simulink model "HillHold"  (R2022b)
settings: Solver=FixedStepDiscrete  StartTime=0.0  StopTime=10.0  FixedStep=0.0001  RelTol=1e-3
undefined symbols (not defined in the file or in its folder): GEAR, MOTORDIR, ParamCfg_HillholdEnable_u16, ParamCfg_HillHoldTime_u16
libraries: simulink x29
settings Model: DataDictionary=MCU_HillHold.sldd  Creator=ZYH  LastModifiedBy=ZYH
settings OptimizationCC: DefaultParameterBehavior=Inlined  EnhancedBackFolding=on  PassReuseOutputArgsAs=Individual arguments  ZeroExternalMemoryAtStartup=off  ZeroInternalMemoryAtStartup=off  OptimizeBlockOrder=speed  DifferentSizesBufferReuse=on  OptimizationCustomize=off  EfficientTunableParamExpr=on
settings DebuggingCC: ParameterTunabilityLossMsg=error
settings SFSimCC: MATLABDynamicMemAlloc=off
settings RTWCC: Description=Embedded Coder  SystemTargetFile=ert.tlc  GenCodeOnly=on  TemplateMakefile=ert_default_tmf
settings CodeAppCC: ForceParamTrailComments=on  IgnoreCustomStorageClasses=off  OperatorAnnotations=on  SimulinkDataObjDesc=on  SFDataObjDesc=on  InsertBlockDesc=on
settings ERTTargetCC: TargetLangStandard=C99 (ISO)  GenerateSampleERTMain=on  InlinedParameterPlacement=NonHierarchical  ERTCustomFileTemplate=example_file_process.tlc

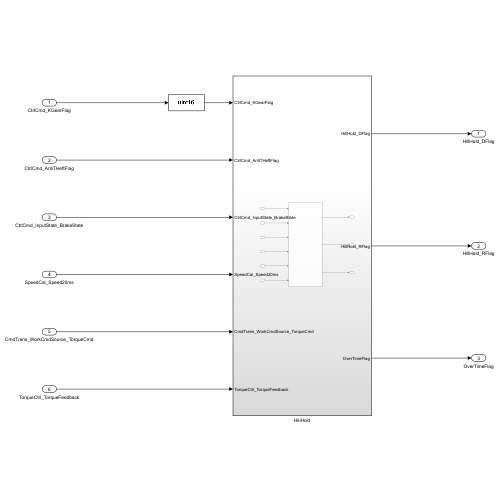
[thumbnail: Simulink's stored preview of the top-level diagram]
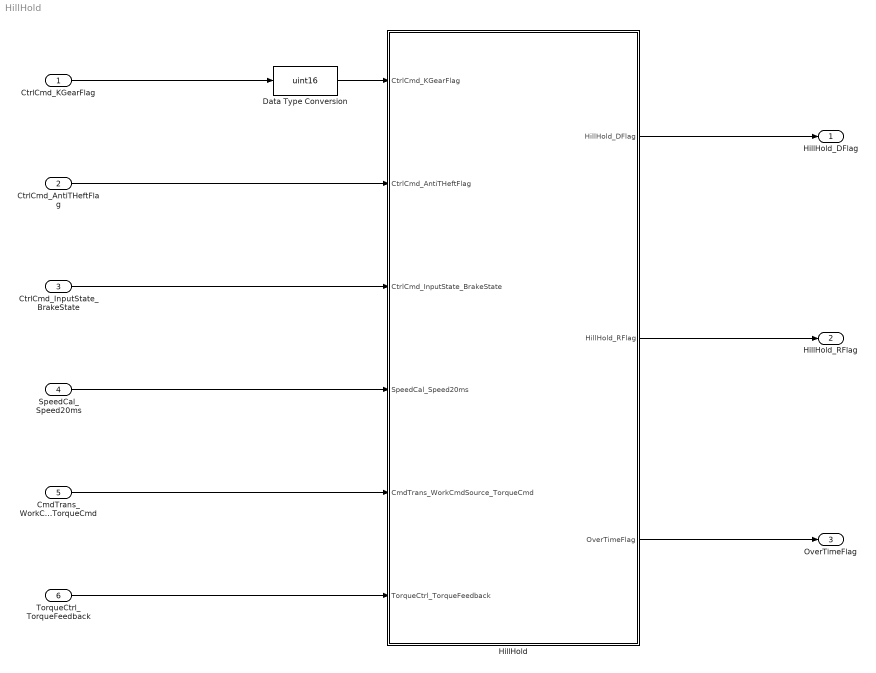
== system HillHold ==
  CtrlCmd_KGearFlag : Inport
  CtrlCmd_AntiTHeftFlag : Inport  Port=2
  CtrlCmd_InputState_BrakeState : Inport  Port=3
  SpeedCal_Speed20ms : Inport  Port=4
  CmdTrans_WorkCmdSource_TorqueCmd : Inport  Port=5
  TorqueCtrl_TorqueFeedback : Inport  Port=6
  Data Type Conversion : DataTypeConversion  OutDataTypeStr=uint16  SaturateOnIntegerOverflow=off  RndMeth=Floor
  HillHold : Subsystem
  HillHold_DFlag : Outport
  HillHold_RFlag : Outport  Port=2
  OverTimeFlag : Outport  Port=3
  wires:
  CtrlCmd_KGearFlag/1 -> Data Type Conversion/1
  CtrlCmd_AntiTHeftFlag/1 -> HillHold/2(CtrlCmd_AntiTHeftFlag)
  Data Type Conversion/1 -> HillHold/1(CtrlCmd_KGearFlag)
  CtrlCmd_InputState_BrakeState/1 -> HillHold/3(CtrlCmd_InputState_BrakeState)
  SpeedCal_Speed20ms/1 -> HillHold/4(SpeedCal_Speed20ms)
  CmdTrans_WorkCmdSource_TorqueCmd/1 -> HillHold/5(CmdTrans_WorkCmdSource_TorqueCmd)
  TorqueCtrl_TorqueFeedback/1 -> HillHold/6(TorqueCtrl_TorqueFeedback)
  HillHold/1(HillHold_DFlag) -> HillHold_DFlag/1
  HillHold/2(HillHold_RFlag) -> HillHold_RFlag/1
  HillHold/3(OverTimeFlag) -> OverTimeFlag/1

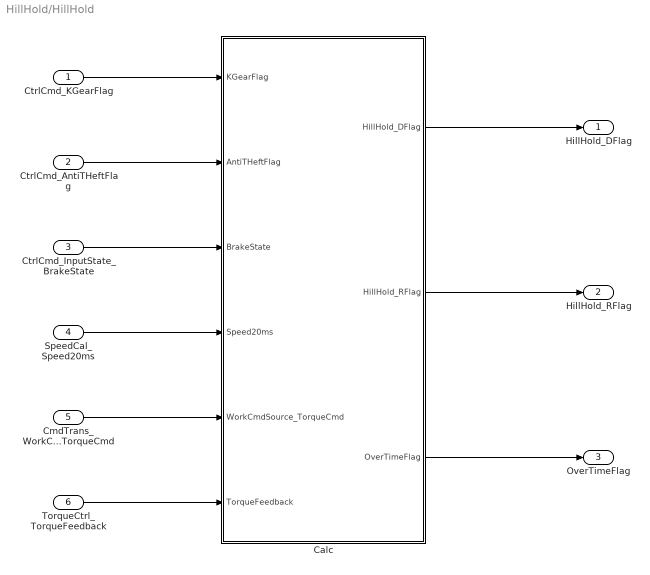
== system HillHold/HillHold ==
  CtrlCmd_KGearFlag : Inport
  CtrlCmd_AntiTHeftFlag : Inport  Port=2
  CtrlCmd_InputState_BrakeState : Inport  Port=3
  SpeedCal_Speed20ms : Inport  Port=4
  CmdTrans_WorkCmdSource_TorqueCmd : Inport  Port=5
  TorqueCtrl_TorqueFeedback : Inport  Port=6
  Calc : Subsystem
  HillHold_DFlag : Outport
  HillHold_RFlag : Outport  Port=2
  OverTimeFlag : Outport  Port=3
  wires:
  CtrlCmd_KGearFlag/1 -> Calc/1(KGearFlag)
  CtrlCmd_AntiTHeftFlag/1 -> Calc/2(AntiTHeftFlag)
  CtrlCmd_InputState_BrakeState/1 -> Calc/3(BrakeState)
  SpeedCal_Speed20ms/1 -> Calc/4(Speed20ms)
  CmdTrans_WorkCmdSource_TorqueCmd/1 -> Calc/5(WorkCmdSource_TorqueCmd)
  TorqueCtrl_TorqueFeedback/1 -> Calc/6(TorqueFeedback)
  Calc/1(HillHold_DFlag) -> HillHold_DFlag/1
  Calc/2(HillHold_RFlag) -> HillHold_RFlag/1
  Calc/3(OverTimeFlag) -> OverTimeFlag/1

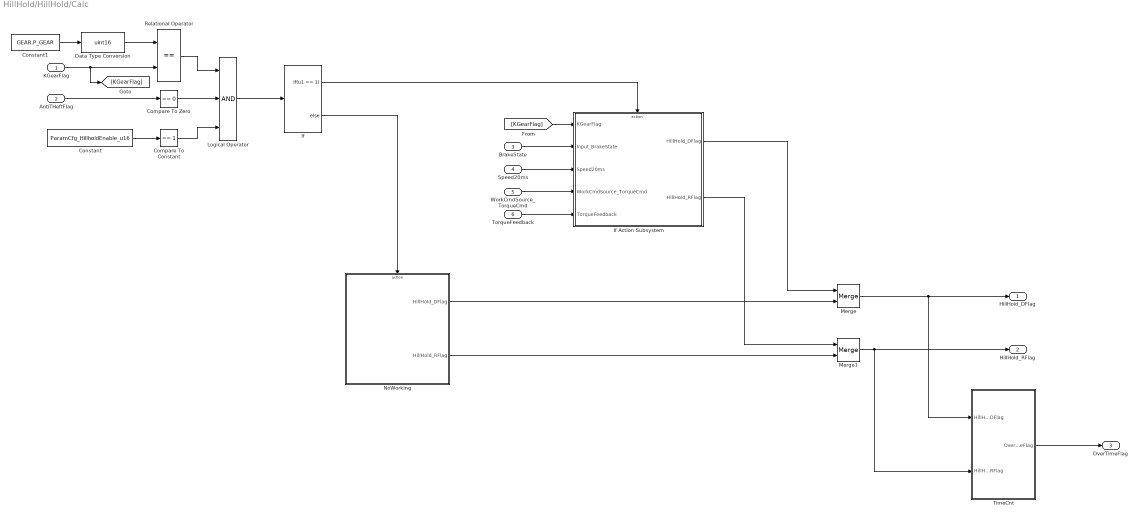
== system HillHold/HillHold/Calc ==
  KGearFlag : Inport
  AntiTHeftFlag : Inport  Port=2
  BrakeState : Inport  Port=3
  Speed20ms : Inport  Port=4
  WorkCmdSource_TorqueCmd : Inport  Port=5
  TorqueFeedback : Inport  Port=6
  Compare To Constant : simulink/Logic and Bit Operations/Compare To Constant  relop===  const=1  OutDataTypeStr=boolean
  Compare To Zero : simulink/Logic and Bit Operations/Compare To Zero  relop===  OutDataTypeStr=boolean
  Constant : Constant  Value=ParamCfg_HillholdEnable_u16  OutDataTypeStr=uint16
  Constant1 : Constant  Value=GEAR.P_GEAR
  Data Type Conversion : DataTypeConversion  OutDataTypeStr=uint16  SaturateOnIntegerOverflow=off  RndMeth=Floor
  If : If  IfExpression=u1 == 1
  If Action Subsystem : Subsystem  TreatAsAtomicUnit=on
  Logical Operator : Logic  Inputs=3  AllPortsSameDT=off  OutDataTypeStr=boolean
  Merge : Merge
  Merge1 : Merge
  NoWorking : Subsystem  TreatAsAtomicUnit=on
  Relational Operator : RelationalOperator  Operator===  OutDataTypeStr=boolean  RndMeth=Simplest  InputSameDT=off
  TimeCnt : Subsystem
  HillHold_DFlag : Outport
  HillHold_RFlag : Outport  Port=2
  OverTimeFlag : Outport  Port=3
  wires:
  KGearFlag/1 -> [KGearFlag], Relational Operator/2
  Constant1/1 -> Data Type Conversion/1
  AntiTHeftFlag/1 -> Compare To Zero/1
  Constant/1 -> Compare To Constant/1
  Relational Operator/1 -> Logical Operator/1
  Compare To Zero/1 -> Logical Operator/2
  Compare To Constant/1 -> Logical Operator/3
  Logical Operator/1 -> If/1
  If/1 -> If Action Subsystem/Action
  If/2 -> NoWorking/Action
  [KGearFlag] -> If Action Subsystem/1(KGearFlag)
  Data Type Conversion/1 -> Relational Operator/1
  BrakeState/1 -> If Action Subsystem/2(Input_BrakeState)
  Speed20ms/1 -> If Action Subsystem/3(Speed20ms)
  WorkCmdSource_TorqueCmd/1 -> If Action Subsystem/4(WorkCmdSource_TorqueCmd)
  TorqueFeedback/1 -> If Action Subsystem/5(TorqueFeedback)
  Merge/1 -> TimeCnt/1(HillHold_DFlag), HillHold_DFlag/1
  Merge1/1 -> TimeCnt/2(HillHold_RFlag), HillHold_RFlag/1
  If Action Subsystem/1(HillHold_DFlag) -> Merge/1
  NoWorking/1(HillHold_DFlag) -> Merge/2
  NoWorking/2(HillHold_RFlag) -> Merge1/2
  If Action Subsystem/2(HillHold_RFlag) -> Merge1/1
  TimeCnt/1(OverTimeFlag) -> OverTimeFlag/1

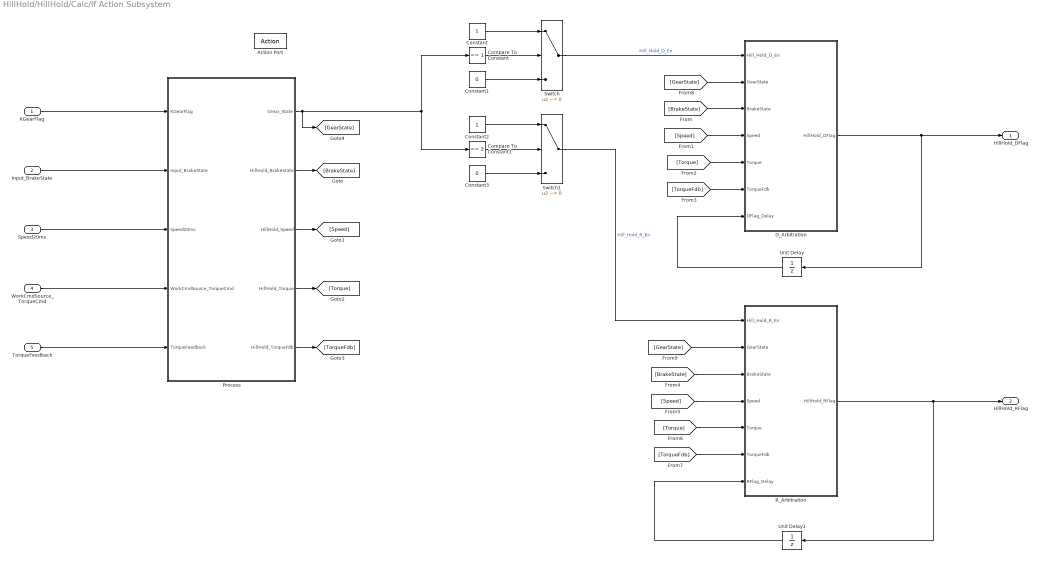
== system HillHold/HillHold/Calc/If Action Subsystem ==
  KGearFlag : Inport
  Input_BrakeState : Inport  Port=2
  Speed20ms : Inport  Port=3
  WorkCmdSource_TorqueCmd : Inport  Port=4
  TorqueFeedback : Inport  Port=5
  Action Port : ActionPort  ActionPortLabel=if(u1 == 1)
  Compare To Constant : simulink/Logic and Bit Operations/Compare To Constant  relop===  const=1  OutDataTypeStr=boolean
  Compare To Constant1 : simulink/Logic and Bit Operations/Compare To Constant  relop===  const=2  OutDataTypeStr=boolean
  Constant : Constant  OutDataTypeStr=uint8
  Constant1 : Constant  Value=0  OutDataTypeStr=uint8
  Constant2 : Constant  OutDataTypeStr=uint8
  Constant3 : Constant  Value=0  OutDataTypeStr=uint8
  D_Arbitration : Subsystem
  Process : Subsystem
  R_Arbitration : Subsystem
  Switch : Switch  Criteria=u2 ~= 0  SaturateOnIntegerOverflow=off  InputSameDT=off
  Switch1 : Switch  Criteria=u2 ~= 0  SaturateOnIntegerOverflow=off  InputSameDT=off
  Unit Delay : UnitDelay  SampleTime=-1  HasFrameUpgradeWarning=on
  Unit Delay1 : UnitDelay  SampleTime=-1  HasFrameUpgradeWarning=on
  HillHold_DFlag : Outport
  HillHold_RFlag : Outport  Port=2
  wires:
  KGearFlag/1 -> Process/1(KGearFlag)
  Input_BrakeState/1 -> Process/2(Input_BrakeState)
  Speed20ms/1 -> Process/3(Speed20ms)
  WorkCmdSource_TorqueCmd/1 -> Process/4(WorkCmdSource_TorqueCmd)
  TorqueFeedback/1 -> Process/5(TorqueFeedback)
  Process/1(Grear_State) -> [GearState], Compare To Constant/1, Compare To Constant1/1
  Compare To Constant/1 -> Switch/2
  Constant/1 -> Switch/1
  Constant1/1 -> Switch/3
  Switch/1 -> D_Arbitration/1(Hill_Hold_D_En)  "Hill_Hold_D_En"
  Compare To Constant1/1 -> Switch1/2
  Constant2/1 -> Switch1/1
  Constant3/1 -> Switch1/3
  Switch1/1 -> R_Arbitration/1(Hill_Hold_R_En)  "Hill_Hold_R_En"
  D_Arbitration/1(HillHold_DFlag) -> Unit Delay/1, HillHold_DFlag/1
  R_Arbitration/1(HillHold_RFlag) -> Unit Delay1/1, HillHold_RFlag/1
  Process/2(HillHold_BrakeState) -> [BrakeState]
  Process/3(HillHold_Speed) -> [Speed]
  Process/4(HillHold_Torque) -> [Torque]
  Process/5(HillHold_TorqueFdb) -> [TorqueFdb]
  [BrakeState] -> D_Arbitration/3(BrakeState)
  [Torque] -> D_Arbitration/5(Torque)
  [TorqueFdb] -> D_Arbitration/6(TorqueFdb)
  [Speed] -> D_Arbitration/4(Speed)
  [Torque] -> R_Arbitration/5(Torque)
  [TorqueFdb] -> R_Arbitration/6(TorqueFdb)
  [BrakeState] -> R_Arbitration/3(BrakeState)
  [Speed] -> R_Arbitration/4(Speed)
  Unit Delay/1 -> D_Arbitration/7(DFlag_Delay)
  [GearState] -> D_Arbitration/2(GearState)
  Unit Delay1/1 -> R_Arbitration/7(RFlag_Delay)
  [GearState] -> R_Arbitration/2(GearState)

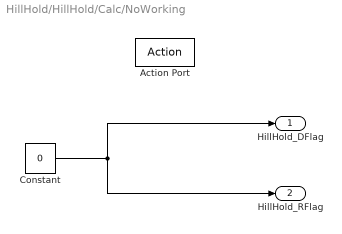
== system HillHold/HillHold/Calc/NoWorking ==
  Action Port : ActionPort  ActionPortLabel=else
  Constant : Constant  Value=0  OutDataTypeStr=uint8
  HillHold_DFlag : Outport
  HillHold_RFlag : Outport  Port=2
  wires:
  Constant/1 -> HillHold_DFlag/1, HillHold_RFlag/1

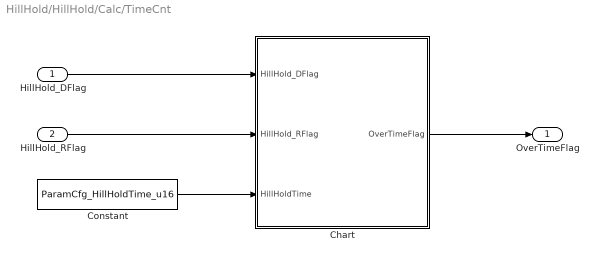
== system HillHold/HillHold/Calc/TimeCnt ==
  HillHold_DFlag : Inport
  HillHold_RFlag : Inport  Port=2
  Chart : Stateflow chart  TreatAsAtomicUnit=on
      settings: PortSchema="{\"entries\":[{\"content\":{\"sides\":[{\"content\":{\"connectorIds\":[\"In2\",\"In1\",\"In3\"]},\"type\":\"ConnectorPlacement.EquallySpacedRectSide\",\"uuid\":\"ad3b6c9c-7775-4671-bd60-29f17afbffc4\"},{\"content\":{\"connectorIds\":[\"Out1\"],\"side\":\"RIGHT\"},\"type\":\"ConnectorPlacement.EquallySpacedRectSide\",\"uuid\":\"3a495722-37f8-4c2a-93d3-d5ac64209b30\"},{\"content\":{\"connectorIds\":[],\"side\":\"TOP\"},\"type\":\"ConnectorPlacement.EquallySpacedRectSide\",\"uuid\":\"2a76a110-b29d-49f8-a37c-690cc675ae55\"},{\"content\":{\"connectorIds\":[],\"side\":\"BOTTOM\"},\"type\":\"ConnectorPlacement.EquallySpacedRectSide\",\"uuid\":\"89755bf0-fe15-44cd-9046-184cf59b0786\"}]},\"type\":\"ConnectorPlacement.EquallySpacedConnector\",\"uuid\":\"915e6b81-f02b-42c3-a3d4-85a899ba8ca8\"}],\"packageUris\":[\"http://schema.mathworks.com/mf0/Connector/R2020b\"],\"version\":\"1.0\"}"
  Constant : Constant  Value=ParamCfg_HillHoldTime_u16
  OverTimeFlag : Outport
  wires:
  HillHold_DFlag/1 -> Chart/2(HillHold_DFlag)
  HillHold_RFlag/1 -> Chart/1(HillHold_RFlag)
  Constant/1 -> Chart/3(HillHoldTime)
  Chart/1(OverTimeFlag) -> OverTimeFlag/1

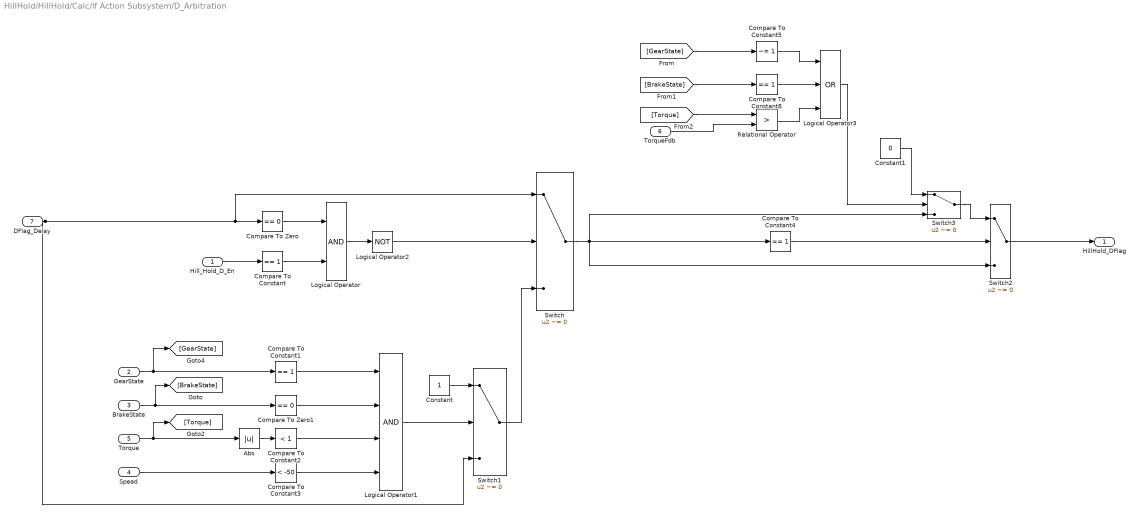
== system HillHold/HillHold/Calc/If Action Subsystem/D_Arbitration ==
  Hill_Hold_D_En : Inport
  GearState : Inport  Port=2
  BrakeState : Inport  Port=3
  Speed : Inport  Port=4
  Torque : Inport  Port=5
  TorqueFdb : Inport  Port=6
  DFlag_Delay : Inport  Port=7
  Abs : Abs  SaturateOnIntegerOverflow=off
  Compare To Constant{,1,4,8} (4 alike) : simulink/Logic and Bit Operations/Compare To Constant  relop===  const=1  OutDataTypeStr=boolean
  Compare To Constant2 : simulink/Logic and Bit Operations/Compare To Constant  relop=<  const=1  OutDataTypeStr=boolean
  Compare To Constant3 : simulink/Logic and Bit Operations/Compare To Constant  relop=<  const=-50  OutDataTypeStr=boolean
  Compare To Constant5 : simulink/Logic and Bit Operations/Compare To Constant  relop=~=  const=1  OutDataTypeStr=boolean
  Compare To Zero : simulink/Logic and Bit Operations/Compare To Zero  relop===  OutDataTypeStr=boolean
  Compare To Zero1 : simulink/Logic and Bit Operations/Compare To Zero  relop===  OutDataTypeStr=boolean
  Constant : Constant  OutDataTypeStr=uint8
  Constant1 : Constant  Value=0  OutDataTypeStr=uint8
  Logical Operator : Logic  AllPortsSameDT=off  OutDataTypeStr=boolean
  Logical Operator1 : Logic  Inputs=4  AllPortsSameDT=off  OutDataTypeStr=boolean
  Logical Operator2 : Logic  Operator=NOT  AllPortsSameDT=off  OutDataTypeStr=boolean
  Logical Operator3 : Logic  Operator=OR  Inputs=3  AllPortsSameDT=off  OutDataTypeStr=boolean
  Relational Operator : RelationalOperator  Operator=>  OutDataTypeStr=boolean  RndMeth=Simplest  InputSameDT=off
  Switch{,1..3} (4 alike) : Switch  Criteria=u2 ~= 0  SaturateOnIntegerOverflow=off  InputSameDT=off
  HillHold_DFlag : Outport
  wires:
  Hill_Hold_D_En/1 -> Compare To Constant/1
  DFlag_Delay/1 -> Switch/1, Compare To Zero/1, Switch1/3
  Compare To Zero/1 -> Logical Operator/1
  Compare To Constant/1 -> Logical Operator/2
  Logical Operator/1 -> Logical Operator2/1
  BrakeState/1 -> Compare To Zero1/1, [BrakeState]
  GearState/1 -> Compare To Constant1/1, [GearState]
  Torque/1 -> Abs/1, [Torque]
  Speed/1 -> Compare To Constant3/1
  Compare To Constant1/1 -> Logical Operator1/1
  Compare To Zero1/1 -> Logical Operator1/2
  Compare To Constant2/1 -> Logical Operator1/3
  Compare To Constant3/1 -> Logical Operator1/4
  Logical Operator1/1 -> Switch1/2
  Constant/1 -> Switch1/1
  Switch1/1 -> Switch/3
  Logical Operator2/1 -> Switch/2
  Switch/1 -> Compare To Constant4/1, Switch3/3, Switch2/3
  Compare To Constant4/1 -> Switch2/2
  [GearState] -> Compare To Constant5/1
  [BrakeState] -> Compare To Constant8/1
  [Torque] -> Relational Operator/1
  TorqueFdb/1 -> Relational Operator/2
  Compare To Constant8/1 -> Logical Operator3/2
  Relational Operator/1 -> Logical Operator3/3
  Compare To Constant5/1 -> Logical Operator3/1
  Logical Operator3/1 -> Switch3/2
  Constant1/1 -> Switch3/1
  Switch3/1 -> Switch2/1
  Switch2/1 -> HillHold_DFlag/1
  Abs/1 -> Compare To Constant2/1

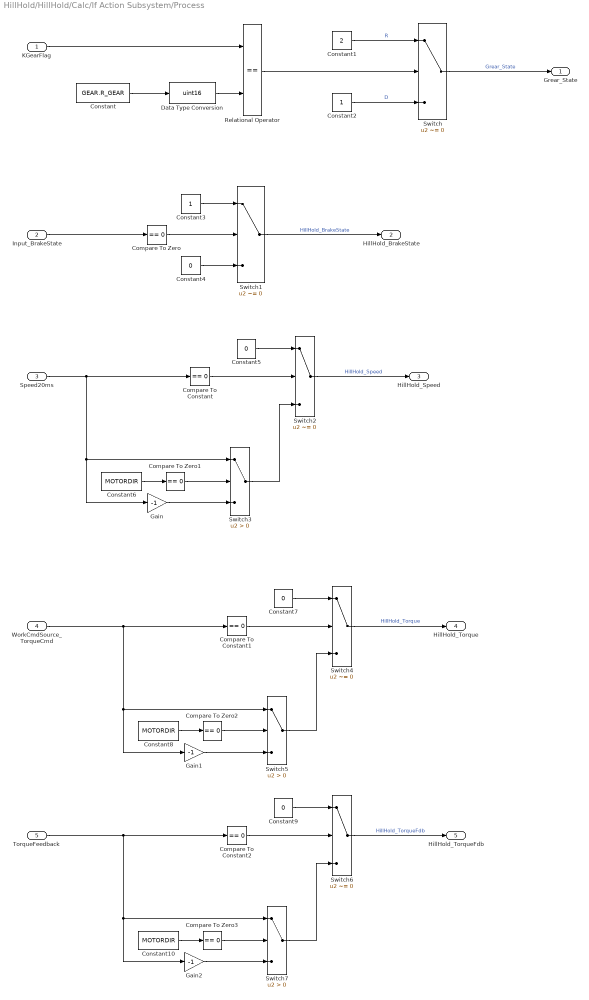
== system HillHold/HillHold/Calc/If Action Subsystem/Process ==
  KGearFlag : Inport
  Input_BrakeState : Inport  Port=2
  Speed20ms : Inport  Port=3
  WorkCmdSource_TorqueCmd : Inport  Port=4
  TorqueFeedback : Inport  Port=5
  Compare To Constant : simulink/Logic and Bit Operations/Compare To Constant  relop===  const=0  OutDataTypeStr=boolean
  Compare To Constant1 : simulink/Logic and Bit Operations/Compare To Constant  relop===  const=0  OutDataTypeStr=boolean
  Compare To Constant2 : simulink/Logic and Bit Operations/Compare To Constant  relop===  const=0  OutDataTypeStr=boolean
  Compare To Zero{,1..3} (4 alike) : simulink/Logic and Bit Operations/Compare To Zero  relop===  OutDataTypeStr=boolean
  Constant : Constant  Value=GEAR.R_GEAR
  Constant1 : Constant  Value=2  OutDataTypeStr=uint8
  Constant10 : Constant  Value=MOTORDIR
  Constant2 : Constant  OutDataTypeStr=uint8
  Constant3 : Constant  OutDataTypeStr=uint8
  Constant4 : Constant  Value=0  OutDataTypeStr=uint8
  Constant5 : Constant  Value=0  OutDataTypeStr=single
  Constant6 : Constant  Value=MOTORDIR
  Constant7 : Constant  Value=0  OutDataTypeStr=single
  Constant8 : Constant  Value=MOTORDIR
  Constant9 : Constant  Value=0  OutDataTypeStr=single
  Data Type Conversion : DataTypeConversion  OutDataTypeStr=uint16  SaturateOnIntegerOverflow=off  RndMeth=Floor
  Gain : Gain  Gain=-1  ParamDataTypeStr=single  OutDataTypeStr=single
  Gain1 : Gain  Gain=-1  ParamDataTypeStr=single  OutDataTypeStr=single
  Gain2 : Gain  Gain=-1  ParamDataTypeStr=single  OutDataTypeStr=single
  Relational Operator : RelationalOperator  Operator===  OutDataTypeStr=boolean  RndMeth=Simplest  InputSameDT=off
  Switch{,1..2,4,6} (5 alike) : Switch  Criteria=u2 ~= 0  SaturateOnIntegerOverflow=off  InputSameDT=off
  Switch3 : Switch  Criteria=u2 > Threshold  SaturateOnIntegerOverflow=off  InputSameDT=off
  Switch5 : Switch  Criteria=u2 > Threshold  SaturateOnIntegerOverflow=off  InputSameDT=off
  Switch7 : Switch  Criteria=u2 > Threshold  SaturateOnIntegerOverflow=off  InputSameDT=off
  Grear_State : Outport
  HillHold_BrakeState : Outport  Port=2
  HillHold_Speed : Outport  Port=3
  HillHold_Torque : Outport  Port=4
  HillHold_TorqueFdb : Outport  Port=5
  wires:
  Compare To Zero3/1 -> Switch7/2
  Compare To Constant2/1 -> Switch6/2
  Switch7/1 -> Switch6/3
  Constant3/1 -> Switch1/1
  Speed20ms/1 -> Switch3/1, Gain/1, Compare To Constant/1
  Switch/1 -> Grear_State/1  "Grear_State"
  Constant9/1 -> Switch6/1
  WorkCmdSource_TorqueCmd/1 -> Switch5/1, Gain1/1, Compare To Constant1/1
  TorqueFeedback/1 -> Switch7/1, Gain2/1, Compare To Constant2/1
  Constant10/1 -> Compare To Zero3/1
  Switch1/1 -> HillHold_BrakeState/1  "HillHold_BrakeState"
  Gain2/1 -> Switch7/3
  Switch6/1 -> HillHold_TorqueFdb/1  "HillHold_TorqueFdb"
  Constant5/1 -> Switch2/1
  Compare To Zero/1 -> Switch1/2
  Switch4/1 -> HillHold_Torque/1  "HillHold_Torque"
  Compare To Zero1/1 -> Switch3/2
  Compare To Constant/1 -> Switch2/2
  Constant/1 -> Data Type Conversion/1
  Data Type Conversion/1 -> Relational Operator/2
  Constant1/1 -> Switch/1  "R"
  Gain1/1 -> Switch5/3
  Constant2/1 -> Switch/3  "D"
  Constant8/1 -> Compare To Zero2/1
  Switch5/1 -> Switch4/3
  Relational Operator/1 -> Switch/2
  Switch2/1 -> HillHold_Speed/1  "HillHold_Speed"
  Gain/1 -> Switch3/3
  Constant4/1 -> Switch1/3
  Switch3/1 -> Switch2/3
  KGearFlag/1 -> Relational Operator/1
  Compare To Constant1/1 -> Switch4/2
  Constant7/1 -> Switch4/1
  Compare To Zero2/1 -> Switch5/2
  Constant6/1 -> Compare To Zero1/1
  Input_BrakeState/1 -> Compare To Zero/1

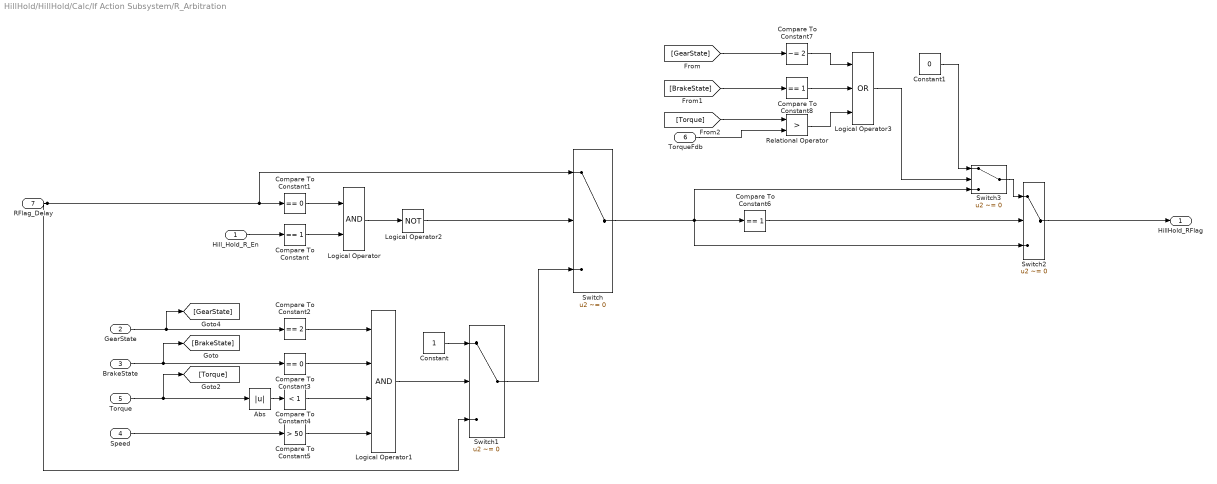
== system HillHold/HillHold/Calc/If Action Subsystem/R_Arbitration ==
  Hill_Hold_R_En : Inport
  GearState : Inport  Port=2
  BrakeState : Inport  Port=3
  Speed : Inport  Port=4
  Torque : Inport  Port=5
  TorqueFdb : Inport  Port=6
  RFlag_Delay : Inport  Port=7
  Abs : Abs  SaturateOnIntegerOverflow=off
  Compare To Constant : simulink/Logic and Bit Operations/Compare To Constant  relop===  const=1  OutDataTypeStr=boolean
  Compare To Constant1 : simulink/Logic and Bit Operations/Compare To Constant  relop===  const=0  OutDataTypeStr=boolean
  Compare To Constant2 : simulink/Logic and Bit Operations/Compare To Constant  relop===  const=2  OutDataTypeStr=boolean
  Compare To Constant3 : simulink/Logic and Bit Operations/Compare To Constant  relop===  const=0  OutDataTypeStr=boolean
  Compare To Constant4 : simulink/Logic and Bit Operations/Compare To Constant  relop=<  const=1  OutDataTypeStr=boolean
  Compare To Constant5 : simulink/Logic and Bit Operations/Compare To Constant  relop=>  const=50  OutDataTypeStr=boolean
  Compare To Constant6 : simulink/Logic and Bit Operations/Compare To Constant  relop===  const=1  OutDataTypeStr=boolean
  Compare To Constant7 : simulink/Logic and Bit Operations/Compare To Constant  relop=~=  const=2  OutDataTypeStr=boolean
  Compare To Constant8 : simulink/Logic and Bit Operations/Compare To Constant  relop===  const=1  OutDataTypeStr=boolean
  Constant : Constant  OutDataTypeStr=uint8
  Constant1 : Constant  Value=0  OutDataTypeStr=uint8
  Logical Operator : Logic  AllPortsSameDT=off  OutDataTypeStr=boolean
  Logical Operator1 : Logic  Inputs=4  AllPortsSameDT=off  OutDataTypeStr=boolean
  Logical Operator2 : Logic  Operator=NOT  AllPortsSameDT=off  OutDataTypeStr=boolean
  Logical Operator3 : Logic  Operator=OR  Inputs=3  AllPortsSameDT=off  OutDataTypeStr=boolean
  Relational Operator : RelationalOperator  Operator=>  OutDataTypeStr=boolean  RndMeth=Simplest  InputSameDT=off
  Switch{,1..3} (4 alike) : Switch  Criteria=u2 ~= 0  SaturateOnIntegerOverflow=off  InputSameDT=off
  HillHold_RFlag : Outport
  wires:
  Hill_Hold_R_En/1 -> Compare To Constant/1
  Logical Operator/1 -> Logical Operator2/1
  Logical Operator2/1 -> Switch/2
  Compare To Constant1/1 -> Logical Operator/1
  Compare To Constant/1 -> Logical Operator/2
  GearState/1 -> Compare To Constant2/1, [GearState]
  BrakeState/1 -> Compare To Constant3/1, [BrakeState]
  Torque/1 -> Abs/1, [Torque]
  Speed/1 -> Compare To Constant5/1
  Compare To Constant2/1 -> Logical Operator1/1
  Compare To Constant3/1 -> Logical Operator1/2
  Compare To Constant4/1 -> Logical Operator1/3
  Compare To Constant5/1 -> Logical Operator1/4
  Logical Operator1/1 -> Switch1/2
  Constant/1 -> Switch1/1
  RFlag_Delay/1 -> Switch/1, Compare To Constant1/1, Switch1/3
  Switch1/1 -> Switch/3
  Switch/1 -> Compare To Constant6/1, Switch3/3, Switch2/3
  Compare To Constant6/1 -> Switch2/2
  Abs/1 -> Compare To Constant4/1
  [BrakeState] -> Compare To Constant8/1
  Compare To Constant7/1 -> Logical Operator3/1
  TorqueFdb/1 -> Relational Operator/2
  [Torque] -> Relational Operator/1
  [GearState] -> Compare To Constant7/1
  Compare To Constant8/1 -> Logical Operator3/2
  Relational Operator/1 -> Logical Operator3/3
  Logical Operator3/1 -> Switch3/2
  Constant1/1 -> Switch3/1
  Switch3/1 -> Switch2/1
  Switch2/1 -> HillHold_RFlag/1

== stateflow chart HillHold/Calc/TimeCnt/Chart ==
  (default) -> (junction 3)
  (junction 3) -> (junction 5) [order 1] : [HillHold_DFlag == true && HillHold_RFlag == true]
  (junction 3) -> (junction 21) [order 2] : {
      | OverTimeFlag = false;
      | TimeCnt = 0;
      | }
  (junction 5) -> (junction 7) : [TimeCnt > HillHoldTime]
  (junction 7) -> (junction 12) [order 1]
  (junction 7) -> (junction 18) [order 2] : {TimeCnt = TimeCnt + 1}
  (junction 12) -> (junction 16) : {
      | TimeCnt = HillHoldTime;
      | OverTimeFlag = true;
      | }
  (junction 18) -> (junction 21)
  (junction 16) -> (junction 18)
  (junction 21) -> (junction 24)
  data: HillHold_RFlag input; HillHold_DFlag input; TimeCnt local uint16 =0; HillHoldTime input; OverTimeFlag output uint8 =0
